simulink library "flocking_lib"  (R2018b)
settings: Solver=VariableStepAuto  StartTime=0.0  StopTime=10.0  RelTol=1e-3
settings Model: Creator=sebbe  LastModifiedBy=Sebastian Green

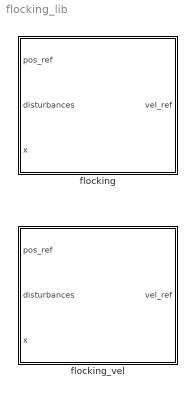
== system flocking_lib ==
  flocking : Subsystem
  flocking_vel : Subsystem

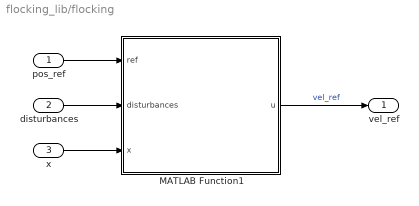
== system flocking_lib/flocking ==
  pos_ref : Inport
  disturbances : Inport  Port=2
  x : Inport  Port=3
  MATLAB Function1 : MATLAB Function  TreatAsAtomicUnit=on
  vel_ref : Outport
  wires:
  pos_ref/1 -> MATLAB Function1/1(ref)
  MATLAB Function1/1(u) -> vel_ref/1  "vel_ref"
  disturbances/1 -> MATLAB Function1/2(disturbances)
  x/1 -> MATLAB Function1/3(x)

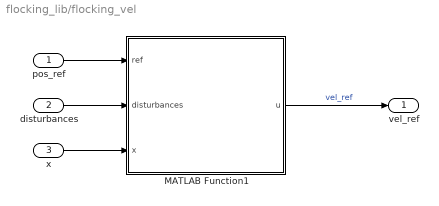
== system flocking_lib/flocking_vel ==
  pos_ref : Inport
  disturbances : Inport  Port=2
  x : Inport  Port=3
  MATLAB Function1 : MATLAB Function  TreatAsAtomicUnit=on
  vel_ref : Outport
  wires:
  x/1 -> MATLAB Function1/3(x)
  disturbances/1 -> MATLAB Function1/2(disturbances)
  MATLAB Function1/1(u) -> vel_ref/1  "vel_ref"
  pos_ref/1 -> MATLAB Function1/1(ref)

== matlab function flocking_lib/flocking/MATLAB Function1 ==
  data: ref input; disturbances input; u output; x input; fc_params parameter
function u = flocking_controller(ref, disturbances, x, fc_params)
% disturbance is 4-C matrix of [x;y;z;dist] for C disturbances
    [~, N] = size(x);
    [~, C] = size(disturbances);
    out = zeros(3, N);
    for n=1:N
        e_r_ref = ref - x(1:3,n); % Position to reference
        e_r_ref_magn = norm(e_r_ref);
        e_r_ref_dir = e_r_ref/e_r_ref_magn;
        %e_rdot_ref = ref - x(4:6,i); % Velocity to reference
        e_rdot_ref = 0 * x(4:6,n); % Not implemented yet
        
        sum_ref_pos = e_r_ref * fc_params.r_ref;
        
        % Limit to +- 1 m/s
        ref_vel_limit = 1;
        %sum_ref_pos(sum_ref_pos>ref_vel_limit) = ref_vel_limit;
        %sum_ref_pos(sum_ref_pos<-ref_vel_limit) = -ref_vel_limit;
        
        sum_ref_vel = e_rdot_ref * fc_params.rdot_ref;
        out(:,n) = out(:,n) + sum_ref_pos + sum_ref_vel;
        
        for c=1:C % Disturbances
            disturbance = disturbances(:,c);
            dist = [x(1:3,n) - disturbance(1:3); disturbance(4)];
            [dir, magn] = calculate_disturbance(dist, 5);
            [~, distance] = calculate_disturbance(dist, 6);
            
            approach_speed = max(0, dot(-dir, x(4:6, n) - [0;0;0]));
            
            n1 = cross(e_r_ref_dir, -dir);
            n2 = cross(e_r_ref_dir, n1);
            n2 = n2/norm(n2) * distance;
            %n2 = n2/norm(n2) * approach_speed/10 * magn;
            
            out_dist = fc_params.r_dist*dir*magn;
            %out(:,n) = out(:,n) + 0.5*out_dist + 0.5*n2 * approach_speed/2;
            out(:,n) = out(:,n) + out_dist;
        end
        
        for j=n+1:N
            e_x = x(:,n) - x(:,j); % Difference between 2 drones in question
            e_r = e_x(1:3); % Position difference
            e_rdot = -e_x(4:6); % Velocity difference
            
            distance = max([norm(e_r), 0.10]); % Absolute distance, 10cm default for first cycle
            
            sum_pos = e_r/distance * fc_params.r_rel;
            sum_vel = e_rdot * fc_params.rdot_rel;
            
            % Push drones "shadowed" by other drones aside to allow tighter
            % formations and more proactive avoidance
            enable_rejection = fc_params.enable_rejection;
            if enable_rejection == 1
                [angle, rej_A, rej_B] = compute_rejections(x(1:3,n) - ref, x(1:3,j) - ref);
                angle_cap = fc_params.angle_cap;
                angle_k = fc_params.angle_k;
                if angle < angle_cap
                    angle_ratio = (angle_cap - angle)/angle_cap;
                    angle_ampl = angle_k*min(1,angle_ratio/distance);
                    rej_A = rej_A*angle_ampl;
                    rej_B = rej_B*angle_ampl;
                else
                    rej_A = rej_A*0;
                    rej_B = rej_B*0;
                end
                out(:,n) = out(:,n) + rej_A;
                out(:,n) = out(:,n) + rej_B;
            end
            
            sum = sum_pos + sum_vel;
            sum = sum/distance;
            
            out(:,n) = out(:,n) + sum;
            out(:,j) = out(:,j) - sum;
        end
    end
	u = out;
end

== matlab function flocking_lib/flocking_vel/MATLAB Function1 ==
  data: ref input; disturbances input; u output; x input; fvc_params parameter
function u = flocking_controller(ref, disturbances, x, fvc_params)
% disturbance is 4-C matrix of [x;y;z;dist] for C disturbances
    [~, N] = size(x);
    [~, C] = size(disturbances);
    out = zeros(3, N);
    for n=1:N
        e_r_ref = ref - x(1:3,n); % Position to reference
        e_r_ref_magn = norm(e_r_ref);
        e_r_ref_dir = e_r_ref/e_r_ref_magn;
        %e_rdot_ref = ref - x(4:6,i); % Velocity to reference
        e_rdot_ref = 0 * x(4:6,n); % Not implemented yet
        
        sum_ref_pos = e_r_ref * fc_params.r_ref;
        
        % Limit to +- 1 m/s
        ref_vel_limit = 1;
        %sum_ref_pos(sum_ref_pos>ref_vel_limit) = ref_vel_limit;
        %sum_ref_pos(sum_ref_pos<-ref_vel_limit) = -ref_vel_limit;
        
        sum_ref_vel = e_rdot_ref * fc_params.rdot_ref;
        out(:,n) = out(:,n) + sum_ref_pos + sum_ref_vel;
        
        for c=1:C % Disturbances
            disturbance = disturbances(:,c);
            dist = [x(1:3,n) - disturbance(1:3); disturbance(4)];
            [dir, magn] = calculate_disturbance(dist, 5);
            [~, distance] = calculate_disturbance(dist, 6);
            
            approach_speed = max(0, dot(-dir, x(4:6, n) - [0;0;0]));
            
            n1 = cross(e_r_ref_dir, -dir);
            n2 = cross(e_r_ref_dir, n1);
            n2 = n2/norm(n2) * distance;
            %n2 = n2/norm(n2) * approach_speed/10 * magn;
            
            out_dist = fc_params.r_dist*dir*magn;
            %out(:,n) = out(:,n) + 0.5*out_dist + 0.5*n2 * approach_speed/2;
            out(:,n) = out(:,n) + out_dist;
        end
        
        for j=n+1:N
            e_x = x(:,n) - x(:,j); % Difference between 2 drones in question
            e_r = e_x(1:3); % Position difference
            e_rdot = -e_x(4:6); % Velocity difference
            
            distance = max([norm(e_r), 0.10]); % Absolute distance, 10cm default for first cycle
            
            sum_pos = e_r * fc_params.r_rel;
            sum_vel = e_rdot * fc_params.rdot_rel;
            
            % Push drones "shadowed" by other drones aside to allow tighter
            % formations and more proactive avoidance
            enable_rejection = 0;
            if enable_rejection == 1
                [angle, rej_A, rej_B] = compute_rejections(x(1:3,n) - ref, x(1:3,j) - ref);
                angle_cap = fc_params.angle_cap;
                angle_k = fc_params.angle_k;
                if angle < angle_cap
                    angle_ratio = (angle_cap - angle)/angle_cap;
                    angle_ampl = angle_k*min(1,angle_ratio/distance);
                    rej_A = rej_A*angle_ampl;
                    rej_B = rej_B*angle_ampl;
                else
                    rej_A = rej_A*0;
                    rej_B = rej_B*0;
                end
                out(:,n) = out(:,n) + rej_A;
                out(:,n) = out(:,n) + rej_B;
            end
            
            sum = sum_pos + sum_vel;
            sum = sum/(distance)^2;
            
            out(:,n) = out(:,n) + sum;
            out(:,j) = out(:,j) - sum;
        end
    end
	u = out;
end
